simulink model "UNIFIER_3DOFsim"  (R2023b)
settings: Solver=VariableStepAuto  StartTime=0  StopTime=t_sim  RelTol=1e-3
InitFcn:
  | UNIFIER_3DOFsim_init
values from neighbouring files (symbols this model uses):
  b = 20.11467    [UNIFIER_LOAD.m]    (also in UNIFIER_LOAD.mat; UNIFIER_LOAD_ROM.m; UNIFIER_LOAD_ROM.mat)
  c = 1.43676    [UNIFIER_LOAD.m]    (also in UNIFIER_LOAD.mat; UNIFIER_LOAD_ROM.m; UNIFIER_LOAD_ROM.mat)
  DEP_inc = -0.0872664625997    [UNIFIER_LOAD.mat]    (also in UNIFIER_ROMdyn.m = deg2rad(-5); UNIFIER_ROMdyn_script.m = deg2rad(-5); UNIFIER_ROMdyn_v2.m = deg2rad(-5); UNIFIER_ROMgen.m = 0.1)
  dp_DEP =     [UNIFIER_LOAD.mat]    (also in UNIFIER_LOAD_ROM.mat)
  dp_FUSE_FIN =     [UNIFIER_LOAD.mat]
  dp_HTU =     [UNIFIER_LOAD.mat]    (also in UNIFIER_LOAD_ROM.mat)
  dp_VTAIL =     [UNIFIER_LOAD.mat]
  dp_VTAIL_INDUCED =     [UNIFIER_LOAD.mat]
  dp_WING_root =     [UNIFIER_LOAD.mat]
  dp_WING_tip =     [UNIFIER_LOAD.mat]
  dumax = [2.09439510239 2.09439510239 2.09439510239 1.0471975512 2 4 2]    [UNIFIER_LOAD.mat]    (also in UNIFIER_LOAD_ROM.mat = [1.0471975512 1.0471975512 1.0471975512 0.174532925199 2 2 2)
  gr = 9.80665    [UNIFIER_LOAD.mat]    (also in UNIFIER_LOAD_ROM.mat)
  m = 7057    [UNIFIER_LOAD.m]    (also in UNIFIER_LOAD.mat; UNIFIER_LOAD_ROM.m; UNIFIER_LOAD_ROM.mat)
  n_prop = 12    [UNIFIER_LOAD.mat]    (also in UNIFIER_ROMdyn.m; UNIFIER_ROMdyn_script.m; UNIFIER_ROMdyn_v2.m)
  prop_d = 1.6    [UNIFIER_LOAD.mat]    (also in UNIFIER_ROMdyn.m; UNIFIER_ROMdyn_script.m; UNIFIER_ROMdyn_v2.m)
  ROMv1 = ROM    [UNIFIER_3DOFsim_init.m]    (also in UNIFIER_ROMgen_subset.m; UNIFIER_ROMgen_v2_subset.m; UNIFIER_ROMgen_v3_subset.m; UNIFIER_ROMgen_v4_subset.m)
  ROMv2 = ROM    [UNIFIER_3DOFsim_init.m]
  ROMv3 = ROM    [UNIFIER_3DOFsim_init.m]
  S = 29.98388    [UNIFIER_LOAD.m]    (also in UNIFIER_LOAD.mat; UNIFIER_LOAD_ROM.m; UNIFIER_LOAD_ROM.mat)
  U_trim = [ustar(3) ... (first row only)    [UNIFIER_3DOFsim_init.m]
  umax = inf    [UNIFIERLanding.m]    (also in UNIFIER_LOAD.mat = [0.436332312999 0.523598775598 0.523598775598 0.436332312999; UNIFIER_LOAD_ROM.mat = [0.436332312999 0.523598775598 0.349065850399 0.436332312999)
  umin = 0    [UNIFIERLanding.m]    (also in UNIFIER_LOAD.mat = [-0.436332312999 -0.523598775598 -0.523598775598 0 0 -1 -0.5; UNIFIER_LOAD_ROM.mat = [-0.436332312999 -0.523598775598 -0.0872664625997 0 0 -1 0])
  Va = sqrt(u^2+w^2)    [ROMcomp.m]    (also in UNIFIERLanding.m = sqrt(x(:,3).^2+x(:,4).^2); UNIFIERLanding_Dynamics_Internal.m = sqrt(X(:,3).^2+X(:,4).^2); UNIFIERLanding_Main.m = sqrt(solution.X(:,3).^2+solution.X(:,4).^2); UNIFIERLanding_trajopt.m = sqrt(solution.X(:,3).^2+solution.X(:,4).^2))
  vtail_nodes = [dp_VTAIL.Xs_LE;     dp_VTAIL.Ys_LE;     dp_VTAIL.Zs_LE]    [UNIFIER_LOAD.m]    (also in UNIFIER_LOAD.mat = [-16.4894695282 -2.83441376686 -2.73765826225 -16.1370849609)
  wing_nodes = [fliplr(dp_WING_tip.LE_Xs),fliplr(dp_WING_root.LE_Xs),dp_WING_root.LE_Xs,dp_WING_tip.LE_Xs;     fliplr(-dp_WING_tip.LE_Ys),fliplr(-dp_WING_root.LE_Ys),dp_WING_root.LE_Ys,dp_WING_tip.LE_Ys;     fliplr(dp_WING_tip.LE_Zs),fliplr(dp_WING_root.LE_Zs),dp_WING_root.LE_Zs,dp_WING_tip.LE_Zs]    [UNIFIER_LOAD.m]    (also in UNIFIER_LOAD.mat = [-7.70795631409 -9.67500019073 -0.98178178072 -7.66801691055)
  x0 = xstar(1)    [UNIFIERLanding.m]    (also in UNIFIER_3DOFsim_init.m; UNIFIER_dynamics.m = x; UNIFIER_trim.m = [Va_target/100; UNIFIER_trim1.m = [Va_target)
  xstar = [0;        0;        -ze_target;        zstar(1)*100;        0;        zstar(2)*100;        0;        zstar(3);        0;        0;        0;        0]    [UNIFIER_trim.m]    (also in UNIFIER_trim0_res.mat = [0 0 -500 55.1327882403 0 -0.446351795968 0 1.36591182427e-0; UNIFIER_trim1.m = [0;        0;        -ze_target;        zstar(1);        0; ; UNIFIER_trim1_res.mat = [0 0 -1219 72.7310470326 0 1.14230710452 0 0.0157060522827 0; UNIFIER_trimHFM.m = [0;        0;        -runconfig.ze;        zstar(1)*100;    )
  xyz_cg = [-8.09,0,-0.2]    [UNIFIER_LOAD.m]    (also in UNIFIER_LOAD.mat = [-8.09 0 -0.2]; UNIFIER_LOAD_ROM.m; UNIFIER_LOAD_ROM.mat = [-8.09 0 -0.2])
  xyz_cg_12 = [-8.09 0 -0.2 -8.09 0 -0.2 -8.09 0 -0.2 -8.09 0 -0.2 ... (36 elements, 3x12)]    [UNIFIER_LOAD.mat]    (also in UNIFIER_LOAD_ROM.mat)
  xyz_DEP = [ -6.9629998	-6.9210000	-6.8660002	-6.8099999	-6.7540002	-6.6999998	-6.6999998	-6.7540002	-6.8099999	-6.8660002	-6.9210000	-6.9629998 ... (first row only)    [UNIFIER_LOAD.m]    (also in UNIFIER_LOAD.mat = [-6.9629998 -10.05 -0.90899998 -6.921 -8.4499998 -0.792 -6.8; UNIFIER_LOAD_ROM.m; UNIFIER_LOAD_ROM.mat = [-6.9629998 -10.05 -0.90899998 -6.921 -8.4499998 -0.792 -6.8)
  z0 = x(1,2)    [UNIFIERLanding.m]    (also in UNIFIER_3DOFsim_init.m = xstar(3); UNIFIER_trim.m = zstar; UNIFIER_trim1.m = zstar; UNIFIER_trimHFM.m = zstar)
undefined symbols (not defined in the file or in its folder): solution
libraries: simulink_extras x17, sharedutil x5, slpidlib x4, aerolibtransform2 x4, dspindex x2, matrix_library x1, shared6dof x1, aerolibatmos2 x1, simulink x1
(part 3 of 4)

== system UNIFIER_3DOFsim/UNIFIER/Aerodynamics/HFM/Aero/VtailForces/VtailForces ==
  rude_defl_nodes : Inport
  alpha_nodes : Inport  Port=2
  beta_nodes : Inport  Port=3
  Interpolation Using Prelookup1 : Interpolation_n-D  NumberOfTableDimensions=4  Table=dp_VTAIL.CFx  NumSelectionDims=1  InternalRulePriority=Speed  TableDataTypeStr=Inherit: Inherit from 'Table data'
      settings: InputPortMap=u0,u1,u2,u3,u4,u5,u6
  Interpolation Using Prelookup2 : Interpolation_n-D  NumberOfTableDimensions=4  Table=dp_VTAIL.CFy  NumSelectionDims=1  InternalRulePriority=Speed  TableDataTypeStr=Inherit: Inherit from 'Table data'
      settings: InputPortMap=u0,u1,u2,u3,u4,u5,u6
  Interpolation Using Prelookup3 : Interpolation_n-D  NumberOfTableDimensions=4  Table=dp_VTAIL.CFz  NumSelectionDims=1  InternalRulePriority=Speed  TableDataTypeStr=Inherit: Inherit from 'Table data'
      settings: InputPortMap=u0,u1,u2,u3,u4,u5,u6
  Interpolation Using Prelookup4 : Interpolation_n-D  NumberOfTableDimensions=4  Table=dp_VTAIL.CMx  NumSelectionDims=1  InternalRulePriority=Speed  TableDataTypeStr=Inherit: Inherit from 'Table data'
      settings: InputPortMap=u0,u1,u2,u3,u4,u5,u6
  Interpolation Using Prelookup5 : Interpolation_n-D  NumberOfTableDimensions=4  Table=dp_VTAIL.CMy  NumSelectionDims=1  InternalRulePriority=Speed  TableDataTypeStr=Inherit: Inherit from 'Table data'
      settings: InputPortMap=u0,u1,u2,u3,u4,u5,u6
  Interpolation Using Prelookup6 : Interpolation_n-D  NumberOfTableDimensions=4  Table=dp_VTAIL.CMz  NumSelectionDims=1  InternalRulePriority=Speed  TableDataTypeStr=Inherit: Inherit from 'Table data'
      settings: InputPortMap=u0,u1,u2,u3,u4,u5,u6
  WingRootPreLookup : Subsystem
  Cx : Outport
  Cy : Outport  Port=2
  Cz : Outport  Port=3
  CMx : Outport  Port=4
  CMy : Outport  Port=5
  CMz : Outport  Port=6
  wires:
  WingRootPreLookup/1(Out1) -> Interpolation Using Prelookup1/1, Interpolation Using Prelookup2/1, Interpolation Using Prelookup3/1, Interpolation Using Prelookup4/1, Interpolation Using Prelookup5/1, Interpolation Using Prelookup6/1
  Interpolation Using Prelookup6/1 -> CMz/1
  Interpolation Using Prelookup5/1 -> CMy/1
  Interpolation Using Prelookup4/1 -> CMx/1
  Interpolation Using Prelookup3/1 -> Cz/1
  Interpolation Using Prelookup2/1 -> Cy/1
  WingRootPreLookup/7(Out5) -> Interpolation Using Prelookup1/7, Interpolation Using Prelookup2/7, Interpolation Using Prelookup3/7, Interpolation Using Prelookup4/7, Interpolation Using Prelookup6/7, Interpolation Using Prelookup5/7
  alpha_nodes/1 -> WingRootPreLookup/2(alpha_nodes)
  beta_nodes/1 -> WingRootPreLookup/3(beta_nodes)
  WingRootPreLookup/2(Out2) -> Interpolation Using Prelookup1/2, Interpolation Using Prelookup2/2, Interpolation Using Prelookup3/2, Interpolation Using Prelookup6/2, Interpolation Using Prelookup5/2, Interpolation Using Prelookup4/2
  WingRootPreLookup/6(Out7) -> Interpolation Using Prelookup1/6, Interpolation Using Prelookup2/6, Interpolation Using Prelookup3/6, Interpolation Using Prelookup4/6, Interpolation Using Prelookup5/6, Interpolation Using Prelookup6/6
  Interpolation Using Prelookup1/1 -> Cx/1
  WingRootPreLookup/5(Out6) -> Interpolation Using Prelookup1/5, Interpolation Using Prelookup2/5, Interpolation Using Prelookup3/5, Interpolation Using Prelookup5/5, Interpolation Using Prelookup6/5, Interpolation Using Prelookup4/5
  WingRootPreLookup/4(Out4) -> Interpolation Using Prelookup1/4, Interpolation Using Prelookup2/4, Interpolation Using Prelookup3/4, Interpolation Using Prelookup4/4, Interpolation Using Prelookup5/4, Interpolation Using Prelookup6/4
  rude_defl_nodes/1 -> WingRootPreLookup/1(rude_defl_nodes)
  WingRootPreLookup/3(Out3) -> Interpolation Using Prelookup1/3, Interpolation Using Prelookup3/3, Interpolation Using Prelookup4/3, Interpolation Using Prelookup5/3, Interpolation Using Prelookup6/3, Interpolation Using Prelookup2/3

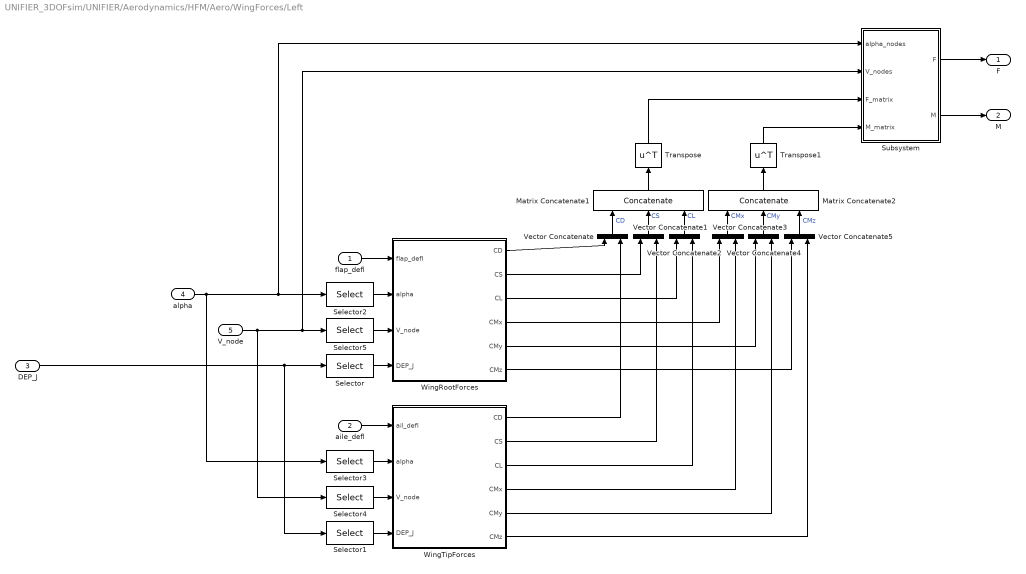
== system UNIFIER_3DOFsim/UNIFIER/Aerodynamics/HFM/Aero/WingForces/Left ==
  flap_defl : Inport
  aile_defl : Inport  Port=2
  DEP_J : Inport  Port=3  PortDimensions=6
  alpha : Inport  Port=4  PortDimensions=7
  V_node : Inport  Port=5  PortDimensions=7
  Matrix Concatenate1 : Concatenate  NumInputs=3  Mode=Multidimensional array  ConcatenateDimension=2
  Matrix Concatenate2 : Concatenate  NumInputs=3  Mode=Multidimensional array  ConcatenateDimension=2
  Selector : Selector  InputPortWidth=6  IndexOptions=Index vector (dialog)  Indices=[1,2,3,4,5]  OutputSizes=1
  Selector1 : Selector  InputPortWidth=6  IndexOptions=Index vector (dialog)  Indices=[5,6]  OutputSizes=1
  Selector2 : Selector  InputPortWidth=7  IndexOptions=Index vector (dialog)  Indices=[1,2,3,4,5]  OutputSizes=1
  Selector3 : Selector  InputPortWidth=7  IndexOptions=Index vector (dialog)  Indices=[6,7]  OutputSizes=1
  Selector4 : Selector  InputPortWidth=7  IndexOptions=Index vector (dialog)  Indices=[6,7]  OutputSizes=1
  Selector5 : Selector  InputPortWidth=7  IndexOptions=Index vector (dialog)  Indices=[1,2,3,4,5]  OutputSizes=1
  Subsystem : Subsystem
  Transpose : Math  Operator=transpose
  Transpose1 : Math  Operator=transpose
  Vector Concatenate{,1..5} (6 alike) : Concatenate
  WingRootForces : Subsystem
  WingTipForces : Subsystem
  F : Outport
  M : Outport  Port=2
  wires:
  Subsystem/2(M) -> M/1
  Subsystem/1(F) -> F/1
  Transpose1/1 -> Subsystem/4(M_matrix)
  Transpose/1 -> Subsystem/3(F_matrix)
  Matrix Concatenate2/1 -> Transpose1/1
  Vector Concatenate5/1 -> Matrix Concatenate2/3  "CMz"
  Vector Concatenate4/1 -> Matrix Concatenate2/2  "CMy"
  Vector Concatenate3/1 -> Matrix Concatenate2/1  "CMx"
  Vector Concatenate2/1 -> Matrix Concatenate1/3  "CL"
  Vector Concatenate/1 -> Matrix Concatenate1/1  "CD"
  Matrix Concatenate1/1 -> Transpose/1
  Vector Concatenate1/1 -> Matrix Concatenate1/2  "CS"
  WingRootForces/5(CMy) -> Vector Concatenate4/1
  WingRootForces/4(CMx) -> Vector Concatenate3/1
  WingRootForces/3(CL) -> Vector Concatenate2/1
  WingRootForces/2(CS) -> Vector Concatenate1/1
  Selector5/1 -> WingRootForces/3(V_node)
  Selector4/1 -> WingTipForces/3(V_node)
  Selector3/1 -> WingTipForces/2(alpha)
  Selector2/1 -> WingRootForces/2(alpha)
  aile_defl/1 -> WingTipForces/1(ail_defl)
  WingTipForces/4(CMx) -> Vector Concatenate3/2
  WingTipForces/5(CMy) -> Vector Concatenate4/2
  WingTipForces/3(CL) -> Vector Concatenate2/2
  WingTipForces/2(CS) -> Vector Concatenate1/2
  WingTipForces/6(CMz) -> Vector Concatenate5/2
  WingTipForces/1(CD) -> Vector Concatenate/2
  WingRootForces/6(CMz) -> Vector Concatenate5/1
  Selector1/1 -> WingTipForces/4(DEP_J)
  WingRootForces/1(CD) -> Vector Concatenate/1
  V_node/1 -> Selector5/1, Subsystem/2(V_nodes), Selector4/1
  Selector/1 -> WingRootForces/4(DEP_J)
  DEP_J/1 -> Selector/1, Selector1/1
  alpha/1 -> Selector3/1, Selector2/1, Subsystem/1(alpha_nodes)
  flap_defl/1 -> WingRootForces/1(flap_defl)

== system UNIFIER_3DOFsim/UNIFIER/Aerodynamics/HFM/Aero/WingForces/Right ==
  flap_defl : Inport
  aile_defl : Inport  Port=2
  DEP_J : Inport  Port=3  PortDimensions=6
  alpha : Inport  Port=4  PortDimensions=7
  V_node : Inport  Port=5  PortDimensions=7
  Matrix Concatenate1 : Concatenate  NumInputs=3  Mode=Multidimensional array  ConcatenateDimension=2
  Matrix Concatenate2 : Concatenate  NumInputs=3  Mode=Multidimensional array  ConcatenateDimension=2
  Selector : Selector  InputPortWidth=6  IndexOptions=Index vector (dialog)  Indices=[1,2,3,4,5]  OutputSizes=1
  Selector1 : Selector  InputPortWidth=6  IndexOptions=Index vector (dialog)  Indices=[5,6]  OutputSizes=1
  Selector2 : Selector  InputPortWidth=7  IndexOptions=Index vector (dialog)  Indices=[1,2,3,4,5]  OutputSizes=1
  Selector3 : Selector  InputPortWidth=7  IndexOptions=Index vector (dialog)  Indices=[6,7]  OutputSizes=1
  Selector4 : Selector  InputPortWidth=7  IndexOptions=Index vector (dialog)  Indices=[6,7]  OutputSizes=1
  Selector5 : Selector  InputPortWidth=7  IndexOptions=Index vector (dialog)  Indices=[1,2,3,4,5]  OutputSizes=1
  Subsystem : Subsystem
  Transpose : Math  Operator=transpose
  Transpose1 : Math  Operator=transpose
  Vector Concatenate{,1..5} (6 alike) : Concatenate
  WingRootForces : Subsystem
  WingTipForces : Subsystem
  F : Outport
  M : Outport  Port=2
  wires:
  Subsystem/2(M) -> M/1
  Subsystem/1(F) -> F/1
  Transpose1/1 -> Subsystem/4(M_matrix)
  Transpose/1 -> Subsystem/3(F_matrix)
  Matrix Concatenate2/1 -> Transpose1/1
  Vector Concatenate5/1 -> Matrix Concatenate2/3  "CMz"
  Vector Concatenate4/1 -> Matrix Concatenate2/2  "CMy"
  Vector Concatenate3/1 -> Matrix Concatenate2/1  "CMx"
  Vector Concatenate2/1 -> Matrix Concatenate1/3  "CL"
  Vector Concatenate/1 -> Matrix Concatenate1/1  "CD"
  Matrix Concatenate1/1 -> Transpose/1
  Vector Concatenate1/1 -> Matrix Concatenate1/2  "CS"
  WingRootForces/5(CMy) -> Vector Concatenate4/1
  WingRootForces/4(CMx) -> Vector Concatenate3/1
  WingRootForces/3(CL) -> Vector Concatenate2/1
  WingRootForces/2(CS) -> Vector Concatenate1/1
  Selector5/1 -> WingRootForces/3(V_node)
  Selector4/1 -> WingTipForces/3(V_node)
  Selector3/1 -> WingTipForces/2(alpha)
  Selector2/1 -> WingRootForces/2(alpha)
  aile_defl/1 -> WingTipForces/1(ail_defl)
  WingTipForces/4(CMx) -> Vector Concatenate3/2
  WingTipForces/5(CMy) -> Vector Concatenate4/2
  WingTipForces/3(CL) -> Vector Concatenate2/2
  WingTipForces/2(CS) -> Vector Concatenate1/2
  WingTipForces/6(CMz) -> Vector Concatenate5/2
  WingTipForces/1(CD) -> Vector Concatenate/2
  WingRootForces/6(CMz) -> Vector Concatenate5/1
  Selector1/1 -> WingTipForces/4(DEP_J)
  WingRootForces/1(CD) -> Vector Concatenate/1
  V_node/1 -> Selector5/1, Subsystem/2(V_nodes), Selector4/1
  Selector/1 -> WingRootForces/4(DEP_J)
  DEP_J/1 -> Selector/1, Selector1/1
  alpha/1 -> Selector3/1, Selector2/1, Subsystem/1(alpha_nodes)
  flap_defl/1 -> WingRootForces/1(flap_defl)

== system UNIFIER_3DOFsim/UNIFIER/Aerodynamics/HFM/Aero/WingForces/Subsystem ==
  DEP_J : Inport
  alpha_nodes : Inport  Port=2
  V_nodes : Inport  Port=3
  Demux1 : Demux  Outputs=2
  Demux2 : Demux  Outputs=2
  Demux3 : Demux  Outputs=2
  Selector : Selector  InputPortWidth=6  IndexOptions=Index vector (dialog)  Indices=[6,5,4,3,2,1]  OutputSizes=1
  Selector1 : Selector  InputPortWidth=7  IndexOptions=Index vector (dialog)  Indices=[7,6,5,4,3,2,1]  OutputSizes=1
  Selector2 : Selector  InputPortWidth=7  IndexOptions=Index vector (dialog)  Indices=[7,6,5,4,3,2,1]  OutputSizes=1
  DEP_J_Left : Outport  PortDimensions=6
  alpha_nodes_Left : Outport  Port=2  PortDimensions=7
  V_nodes_Left : Outport  Port=3  PortDimensions=7
  DEP_J_Right : Outport  Port=4  PortDimensions=6
  alpha_nodes_Right : Outport  Port=5  PortDimensions=7
  V_nodes_Right : Outport  Port=6  PortDimensions=7
  wires:
  Demux3/2 -> V_nodes_Right/1
  V_nodes/1 -> Demux3/1
  Selector2/1 -> V_nodes_Left/1
  Demux3/1 -> Selector2/1
  Demux1/1 -> Selector1/1
  Demux1/2 -> alpha_nodes_Right/1
  alpha_nodes/1 -> Demux1/1
  Selector1/1 -> alpha_nodes_Left/1
  Selector/1 -> DEP_J_Left/1
  DEP_J/1 -> Demux2/1
  Demux2/1 -> Selector/1
  Demux2/2 -> DEP_J_Right/1

== system UNIFIER_3DOFsim/UNIFIER/Aerodynamics/HFM/Aero/FinFuselageForces/Subsystem1/Subsystem ==
  beta : Inport
  alpha : Inport  Port=2
  Prelookup : PreLookup  BreakpointsData=dp_FUSE_FIN.beta  IndexSearchMethod=Linear search  BeginIndexSearchUsingPreviousIndexResult=on  ExtrapMethod=Linear
  Prelookup1 : PreLookup  BreakpointsData=dp_FUSE_FIN.aoa  IndexSearchMethod=Linear search  BeginIndexSearchUsingPreviousIndexResult=on  ExtrapMethod=Linear
  Out1 : Outport
  Out2 : Outport  Port=2
  Out3 : Outport  Port=3
  Out4 : Outport  Port=4
  wires:
  Prelookup/2 -> Out2/1
  Prelookup1/2 -> Out4/1
  Prelookup1/1 -> Out3/1
  beta/1 -> Prelookup/1
  alpha/1 -> Prelookup1/1
  Prelookup/1 -> Out1/1

== system UNIFIER_3DOFsim/UNIFIER/Aerodynamics/HFM/Aero/VtailForces/Subsystem/CrossProduct1 ==
  r : Inport  Partition=on  PartitionDimension=2  PartitionWidth=1  PartitionOffset=0
  F : Inport  Port=2  Partition=on  PartitionDimension=2  PartitionWidth=1  PartitionOffset=0
  3x3 Cross Product : sharedutil/3x3 Cross Product  aMode=aMode
  CG : Constant  Value=xyz_cg
  Cast : DataTypeConversion  OutDataTypeStr=single  SaturateOnIntegerOverflow=off  RndMeth=Floor
  For Each : ForEach  DisableCoverage=on  SpecifiedNumIters=16
  Minus : Sum  Inputs=+-
  M : Outport  ConcatenationDimension=2
  wires:
  Cast/1 -> Minus/2
  Minus/1 -> 3x3 Cross Product/1
  CG/1 -> Cast/1
  3x3 Cross Product/1 -> M/1
  r/1 -> Minus/1
  F/1 -> 3x3 Cross Product/2

== system UNIFIER_3DOFsim/UNIFIER/Aerodynamics/HFM/Aero/VtailForces/VtailForces/WingRootPreLookup ==
  rude_defl_nodes : Inport
  alpha_nodes : Inport  Port=2
  beta_nodes : Inport  Port=3
  Constant8 : Constant  Value=0:15
  Prelookup : PreLookup  BreakpointsData=dp_VTAIL.rude_defl  IndexSearchMethod=Linear search  BeginIndexSearchUsingPreviousIndexResult=on  ExtrapMethod=Linear
  Prelookup1 : PreLookup  BreakpointsData=dp_VTAIL.alphas  IndexSearchMethod=Linear search  BeginIndexSearchUsingPreviousIndexResult=on  ExtrapMethod=Linear
  Prelookup2 : PreLookup  BreakpointsData=dp_VTAIL.betas  IndexSearchMethod=Linear search  BeginIndexSearchUsingPreviousIndexResult=on  ExtrapMethod=Linear
  Out1 : Outport
  Out2 : Outport  Port=2
  Out3 : Outport  Port=3
  Out4 : Outport  Port=4
  Out6 : Outport  Port=5
  Out7 : Outport  Port=6
  Out5 : Outport  Port=7
  wires:
  Prelookup2/2 -> Out7/1
  Prelookup2/1 -> Out6/1
  beta_nodes/1 -> Prelookup2/1
  rude_defl_nodes/1 -> Prelookup/1
  Prelookup1/1 -> Out3/1
  alpha_nodes/1 -> Prelookup1/1
  Prelookup/2 -> Out2/1
  Prelookup1/2 -> Out4/1
  Constant8/1 -> Out5/1
  Prelookup/1 -> Out1/1

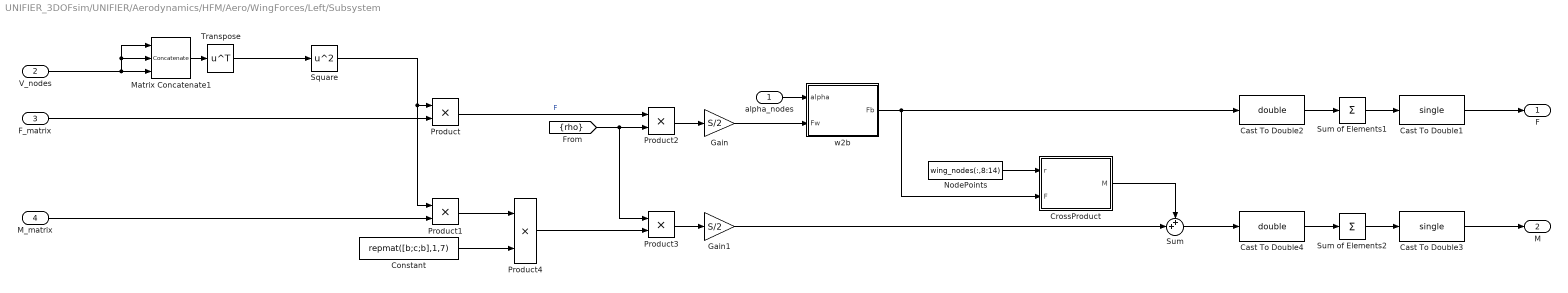
== system UNIFIER_3DOFsim/UNIFIER/Aerodynamics/HFM/Aero/WingForces/Left/Subsystem ==
  alpha_nodes : Inport
  V_nodes : Inport  Port=2
  F_matrix : Inport  Port=3
  M_matrix : Inport  Port=4
  Cast To Double1 : DataTypeConversion  OutDataTypeStr=single  SaturateOnIntegerOverflow=off  RndMeth=Floor
  Cast To Double2 : DataTypeConversion  OutDataTypeStr=double  SaturateOnIntegerOverflow=off  RndMeth=Floor
  Cast To Double3 : DataTypeConversion  OutDataTypeStr=single  SaturateOnIntegerOverflow=off  RndMeth=Floor
  Cast To Double4 : DataTypeConversion  OutDataTypeStr=double  SaturateOnIntegerOverflow=off  RndMeth=Floor
  Constant : Constant  Value=repmat([b;c;b],1,7)
  CrossProduct : Subsystem  TreatAsAtomicUnit=on
  Gain : Gain  Gain=S/2
  Gain1 : Gain  Gain=S/2
  Matrix Concatenate1 : Concatenate  NumInputs=3  Mode=Multidimensional array  ConcatenateDimension=2
  NodePoints : Constant  Value=wing_nodes(:,8:14)
  Product{,1..4} (5 alike) : Product
  Square : Math  Operator=square
  Sum : Sum  Inputs=++|
  Sum of Elements1 : Sum  Inputs=+  CollapseMode=Specified dimension  CollapseDim=2
  Sum of Elements2 : Sum  Inputs=+  CollapseMode=Specified dimension  CollapseDim=2
  Transpose : Math  Operator=transpose
  w2b : Subsystem  TreatAsAtomicUnit=on
  F : Outport
  M : Outport  Port=2
  wires:
  Cast To Double3/1 -> M/1
  Sum/1 -> Cast To Double4/1
  Cast To Double4/1 -> Sum of Elements2/1
  Sum of Elements2/1 -> Cast To Double3/1
  Sum of Elements1/1 -> Cast To Double1/1
  Cast To Double2/1 -> Sum of Elements1/1
  alpha_nodes/1 -> w2b/1(alpha)
  Gain/1 -> w2b/2(Fw)
  Cast To Double1/1 -> F/1
  CrossProduct/1(M) -> Sum/1
  NodePoints/1 -> CrossProduct/1(r)
  w2b/1(Fb) -> CrossProduct/2(F), Cast To Double2/1
  Square/1 -> Product/1, Product1/1
  Matrix Concatenate1/1 -> Transpose/1
  Transpose/1 -> Square/1
  V_nodes/1 -> Matrix Concatenate1/3, Matrix Concatenate1/2, Matrix Concatenate1/1
  Product/1 -> Product2/1  "F"
  Gain1/1 -> Sum/2
  Product1/1 -> Product4/1
  M_matrix/1 -> Product1/2
  Product4/1 -> Product3/2
  Constant/1 -> Product4/2
  Product3/1 -> Gain1/1
  [rho] -> Product2/2, Product3/1
  F_matrix/1 -> Product/2
  Product2/1 -> Gain/1

== system UNIFIER_3DOFsim/UNIFIER/Aerodynamics/HFM/Aero/WingForces/Left/WingRootForces ==
  flap_defl : Inport
  alpha : Inport  Port=2
  V_node : Inport  Port=3
  DEP_J : Inport  Port=4
  Interpolation Using Prelookup1 : Interpolation_n-D  NumberOfTableDimensions=5  Table=dp_WING_root.CD  ExtrapMethod=Clip  ValidIndexMayReachLast=on  NumSelectionDims=1  InternalRulePriority=Speed  TableDataTypeStr=Inherit: Inherit from 'Table data'
      settings: InputPortMap=u0,u1,u2,u3,u4,u5,u6,u7,u8
  Interpolation Using Prelookup2 : Interpolation_n-D  NumberOfTableDimensions=5  Table=dp_WING_root.CS  ExtrapMethod=Clip  ValidIndexMayReachLast=on  NumSelectionDims=1  InternalRulePriority=Speed  TableDataTypeStr=Inherit: Inherit from 'Table data'
      settings: InputPortMap=u0,u1,u2,u3,u4,u5,u6,u7,u8
  Interpolation Using Prelookup3 : Interpolation_n-D  NumberOfTableDimensions=5  Table=dp_WING_root.CL  ExtrapMethod=Clip  ValidIndexMayReachLast=on  NumSelectionDims=1  InternalRulePriority=Speed  TableDataTypeStr=Inherit: Inherit from 'Table data'
      settings: InputPortMap=u0,u1,u2,u3,u4,u5,u6,u7,u8
  Interpolation Using Prelookup4 : Interpolation_n-D  NumberOfTableDimensions=5  Table=dp_WING_root.CMx  ExtrapMethod=Clip  ValidIndexMayReachLast=on  NumSelectionDims=1  InternalRulePriority=Speed  TableDataTypeStr=Inherit: Inherit from 'Table data'
      settings: InputPortMap=u0,u1,u2,u3,u4,u5,u6,u7,u8
  Interpolation Using Prelookup5 : Interpolation_n-D  NumberOfTableDimensions=5  Table=dp_WING_root.CMy  ExtrapMethod=Clip  ValidIndexMayReachLast=on  NumSelectionDims=1  InternalRulePriority=Speed  TableDataTypeStr=Inherit: Inherit from 'Table data'
      settings: InputPortMap=u0,u1,u2,u3,u4,u5,u6,u7,u8
  Interpolation Using Prelookup6 : Interpolation_n-D  NumberOfTableDimensions=5  Table=dp_WING_root.CMz  ExtrapMethod=Clip  ValidIndexMayReachLast=on  NumSelectionDims=1  InternalRulePriority=Speed  TableDataTypeStr=Inherit: Inherit from 'Table data'
      settings: InputPortMap=u0,u1,u2,u3,u4,u5,u6,u7,u8
  WingRootPreLookup : Subsystem
  CD : Outport
  CS : Outport  Port=2
  CL : Outport  Port=3
  CMx : Outport  Port=4
  CMy : Outport  Port=5
  CMz : Outport  Port=6
  wires:
  Interpolation Using Prelookup6/1 -> CMz/1
  Interpolation Using Prelookup5/1 -> CMy/1
  Interpolation Using Prelookup4/1 -> CMx/1
  Interpolation Using Prelookup3/1 -> CL/1
  Interpolation Using Prelookup2/1 -> CS/1
  alpha/1 -> WingRootPreLookup/2(alpha)
  V_node/1 -> WingRootPreLookup/3(V_node)
  DEP_J/1 -> WingRootPreLookup/4(DEP_J)
  WingRootPreLookup/2(Out2) -> Interpolation Using Prelookup1/2, Interpolation Using Prelookup2/2, Interpolation Using Prelookup3/2, Interpolation Using Prelookup4/2, Interpolation Using Prelookup5/2, Interpolation Using Prelookup6/2
  WingRootPreLookup/6(Out7) -> Interpolation Using Prelookup1/6, Interpolation Using Prelookup2/6, Interpolation Using Prelookup3/6, Interpolation Using Prelookup4/6, Interpolation Using Prelookup5/6, Interpolation Using Prelookup6/6
  Interpolation Using Prelookup1/1 -> CD/1
  WingRootPreLookup/5(Out6) -> Interpolation Using Prelookup2/5, Interpolation Using Prelookup3/5, Interpolation Using Prelookup4/5, Interpolation Using Prelookup5/5, Interpolation Using Prelookup6/5, Interpolation Using Prelookup1/5
  WingRootPreLookup/4(Out4) -> Interpolation Using Prelookup1/4, Interpolation Using Prelookup2/4, Interpolation Using Prelookup3/4, Interpolation Using Prelookup4/4, Interpolation Using Prelookup5/4, Interpolation Using Prelookup6/4
  flap_defl/1 -> WingRootPreLookup/1(flap_defl)
  WingRootPreLookup/7(Out8) -> Interpolation Using Prelookup2/7, Interpolation Using Prelookup3/7, Interpolation Using Prelookup4/7, Interpolation Using Prelookup6/7, Interpolation Using Prelookup5/7, Interpolation Using Prelookup1/7
  WingRootPreLookup/1(Out1) -> Interpolation Using Prelookup1/1, Interpolation Using Prelookup2/1, Interpolation Using Prelookup3/1, Interpolation Using Prelookup4/1, Interpolation Using Prelookup5/1, Interpolation Using Prelookup6/1
  WingRootPreLookup/8(Out9) -> Interpolation Using Prelookup1/8, Interpolation Using Prelookup2/8, Interpolation Using Prelookup3/8, Interpolation Using Prelookup4/8, Interpolation Using Prelookup5/8, Interpolation Using Prelookup6/8
  WingRootPreLookup/3(Out3) -> Interpolation Using Prelookup1/3, Interpolation Using Prelookup2/3, Interpolation Using Prelookup3/3, Interpolation Using Prelookup4/3, Interpolation Using Prelookup5/3, Interpolation Using Prelookup6/3
  WingRootPreLookup/9(Out5) -> Interpolation Using Prelookup1/9, Interpolation Using Prelookup2/9, Interpolation Using Prelookup3/9, Interpolation Using Prelookup4/9, Interpolation Using Prelookup5/9, Interpolation Using Prelookup6/9

== system UNIFIER_3DOFsim/UNIFIER/Aerodynamics/HFM/Aero/WingForces/Left/WingTipForces ==
  ail_defl : Inport
  alpha : Inport  Port=2
  V_node : Inport  Port=3
  DEP_J : Inport  Port=4
  Interpolation Using Prelookup1 : Interpolation_n-D  NumberOfTableDimensions=5  Table=dp_WING_tip.CD  ExtrapMethod=Clip  ValidIndexMayReachLast=on  NumSelectionDims=1  InternalRulePriority=Speed  TableDataTypeStr=Inherit: Inherit from 'Table data'
      settings: InputPortMap=u0,u1,u2,u3,u4,u5,u6,u7,u8
  Interpolation Using Prelookup2 : Interpolation_n-D  NumberOfTableDimensions=5  Table=dp_WING_tip.CS  ExtrapMethod=Clip  ValidIndexMayReachLast=on  NumSelectionDims=1  InternalRulePriority=Speed  TableDataTypeStr=Inherit: Inherit from 'Table data'
      settings: InputPortMap=u0,u1,u2,u3,u4,u5,u6,u7,u8
  Interpolation Using Prelookup3 : Interpolation_n-D  NumberOfTableDimensions=5  Table=dp_WING_tip.CL  ExtrapMethod=Clip  ValidIndexMayReachLast=on  NumSelectionDims=1  InternalRulePriority=Speed  TableDataTypeStr=Inherit: Inherit from 'Table data'
      settings: InputPortMap=u0,u1,u2,u3,u4,u5,u6,u7,u8
  Interpolation Using Prelookup4 : Interpolation_n-D  NumberOfTableDimensions=5  Table=dp_WING_tip.CMx  ExtrapMethod=Clip  ValidIndexMayReachLast=on  NumSelectionDims=1  InternalRulePriority=Speed  TableDataTypeStr=Inherit: Inherit from 'Table data'
      settings: InputPortMap=u0,u1,u2,u3,u4,u5,u6,u7,u8
  Interpolation Using Prelookup5 : Interpolation_n-D  NumberOfTableDimensions=5  Table=dp_WING_tip.CMy  ExtrapMethod=Clip  ValidIndexMayReachLast=on  NumSelectionDims=1  InternalRulePriority=Speed  TableDataTypeStr=Inherit: Inherit from 'Table data'
      settings: InputPortMap=u0,u1,u2,u3,u4,u5,u6,u7,u8
  Interpolation Using Prelookup6 : Interpolation_n-D  NumberOfTableDimensions=5  Table=dp_WING_tip.CMz  ExtrapMethod=Clip  ValidIndexMayReachLast=on  NumSelectionDims=1  InternalRulePriority=Speed  TableDataTypeStr=Inherit: Inherit from 'Table data'
      settings: InputPortMap=u0,u1,u2,u3,u4,u5,u6,u7,u8
  WingRootPreLookup : Subsystem
  CD : Outport
  CS : Outport  Port=2
  CL : Outport  Port=3
  CMx : Outport  Port=4
  CMy : Outport  Port=5
  CMz : Outport  Port=6
  wires:
  Interpolation Using Prelookup6/1 -> CMz/1
  Interpolation Using Prelookup5/1 -> CMy/1
  Interpolation Using Prelookup4/1 -> CMx/1
  Interpolation Using Prelookup3/1 -> CL/1
  Interpolation Using Prelookup2/1 -> CS/1
  alpha/1 -> WingRootPreLookup/2(alpha)
  V_node/1 -> WingRootPreLookup/3(V_node)
  DEP_J/1 -> WingRootPreLookup/4(DEP_J)
  WingRootPreLookup/2(Out2) -> Interpolation Using Prelookup1/2, Interpolation Using Prelookup2/2, Interpolation Using Prelookup3/2, Interpolation Using Prelookup4/2, Interpolation Using Prelookup5/2, Interpolation Using Prelookup6/2
  WingRootPreLookup/6(Out7) -> Interpolation Using Prelookup1/6, Interpolation Using Prelookup2/6, Interpolation Using Prelookup3/6, Interpolation Using Prelookup4/6, Interpolation Using Prelookup5/6, Interpolation Using Prelookup6/6
  Interpolation Using Prelookup1/1 -> CD/1
  WingRootPreLookup/5(Out6) -> Interpolation Using Prelookup2/5, Interpolation Using Prelookup3/5, Interpolation Using Prelookup4/5, Interpolation Using Prelookup5/5, Interpolation Using Prelookup6/5, Interpolation Using Prelookup1/5
  WingRootPreLookup/4(Out4) -> Interpolation Using Prelookup1/4, Interpolation Using Prelookup2/4, Interpolation Using Prelookup3/4, Interpolation Using Prelookup4/4, Interpolation Using Prelookup5/4, Interpolation Using Prelookup6/4
  ail_defl/1 -> WingRootPreLookup/1(ail_defl)
  WingRootPreLookup/7(Out8) -> Interpolation Using Prelookup1/7, Interpolation Using Prelookup2/7, Interpolation Using Prelookup3/7, Interpolation Using Prelookup4/7, Interpolation Using Prelookup6/7, Interpolation Using Prelookup5/7
  WingRootPreLookup/1(Out1) -> Interpolation Using Prelookup1/1, Interpolation Using Prelookup2/1, Interpolation Using Prelookup3/1, Interpolation Using Prelookup4/1, Interpolation Using Prelookup5/1, Interpolation Using Prelookup6/1
  WingRootPreLookup/8(Out9) -> Interpolation Using Prelookup1/8, Interpolation Using Prelookup2/8, Interpolation Using Prelookup3/8, Interpolation Using Prelookup4/8, Interpolation Using Prelookup5/8, Interpolation Using Prelookup6/8
  WingRootPreLookup/3(Out3) -> Interpolation Using Prelookup1/3, Interpolation Using Prelookup2/3, Interpolation Using Prelookup3/3, Interpolation Using Prelookup4/3, Interpolation Using Prelookup5/3, Interpolation Using Prelookup6/3
  WingRootPreLookup/9(Out5) -> Interpolation Using Prelookup1/9, Interpolation Using Prelookup2/9, Interpolation Using Prelookup3/9, Interpolation Using Prelookup4/9, Interpolation Using Prelookup5/9, Interpolation Using Prelookup6/9

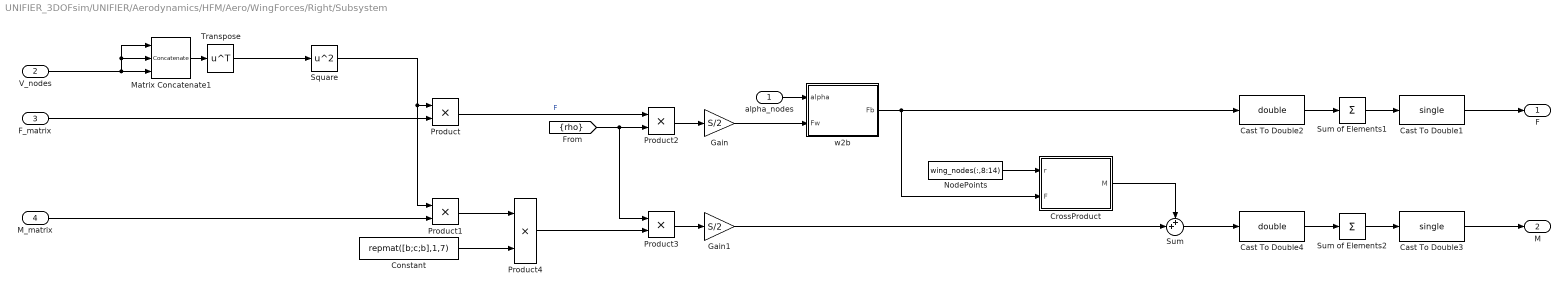
== system UNIFIER_3DOFsim/UNIFIER/Aerodynamics/HFM/Aero/WingForces/Right/Subsystem ==
  alpha_nodes : Inport
  V_nodes : Inport  Port=2
  F_matrix : Inport  Port=3
  M_matrix : Inport  Port=4
  Cast To Double1 : DataTypeConversion  OutDataTypeStr=single  SaturateOnIntegerOverflow=off  RndMeth=Floor
  Cast To Double2 : DataTypeConversion  OutDataTypeStr=double  SaturateOnIntegerOverflow=off  RndMeth=Floor
  Cast To Double3 : DataTypeConversion  OutDataTypeStr=single  SaturateOnIntegerOverflow=off  RndMeth=Floor
  Cast To Double4 : DataTypeConversion  OutDataTypeStr=double  SaturateOnIntegerOverflow=off  RndMeth=Floor
  Constant : Constant  Value=repmat([b;c;b],1,7)
  CrossProduct : Subsystem  TreatAsAtomicUnit=on
  Gain : Gain  Gain=S/2
  Gain1 : Gain  Gain=S/2
  Matrix Concatenate1 : Concatenate  NumInputs=3  Mode=Multidimensional array  ConcatenateDimension=2
  NodePoints : Constant  Value=wing_nodes(:,8:14)
  Product{,1..4} (5 alike) : Product
  Square : Math  Operator=square
  Sum : Sum  Inputs=++|
  Sum of Elements1 : Sum  Inputs=+  CollapseMode=Specified dimension  CollapseDim=2
  Sum of Elements2 : Sum  Inputs=+  CollapseMode=Specified dimension  CollapseDim=2
  Transpose : Math  Operator=transpose
  w2b : Subsystem  TreatAsAtomicUnit=on
  F : Outport
  M : Outport  Port=2
  wires:
  Cast To Double3/1 -> M/1
  Sum/1 -> Cast To Double4/1
  Cast To Double4/1 -> Sum of Elements2/1
  Sum of Elements2/1 -> Cast To Double3/1
  Sum of Elements1/1 -> Cast To Double1/1
  Cast To Double2/1 -> Sum of Elements1/1
  alpha_nodes/1 -> w2b/1(alpha)
  Gain/1 -> w2b/2(Fw)
  Cast To Double1/1 -> F/1
  CrossProduct/1(M) -> Sum/1
  NodePoints/1 -> CrossProduct/1(r)
  w2b/1(Fb) -> CrossProduct/2(F), Cast To Double2/1
  Square/1 -> Product/1, Product1/1
  Matrix Concatenate1/1 -> Transpose/1
  Transpose/1 -> Square/1
  V_nodes/1 -> Matrix Concatenate1/3, Matrix Concatenate1/2, Matrix Concatenate1/1
  Product/1 -> Product2/1  "F"
  Gain1/1 -> Sum/2
  Product1/1 -> Product4/1
  M_matrix/1 -> Product1/2
  Product4/1 -> Product3/2
  Constant/1 -> Product4/2
  Product3/1 -> Gain1/1
  [rho] -> Product2/2, Product3/1
  F_matrix/1 -> Product/2
  Product2/1 -> Gain/1

== system UNIFIER_3DOFsim/UNIFIER/Aerodynamics/HFM/Aero/WingForces/Right/WingRootForces ==
  flap_defl : Inport
  alpha : Inport  Port=2
  V_node : Inport  Port=3
  DEP_J : Inport  Port=4
  Interpolation Using Prelookup1 : Interpolation_n-D  NumberOfTableDimensions=5  Table=dp_WING_root.CD  ExtrapMethod=Clip  ValidIndexMayReachLast=on  NumSelectionDims=1  InternalRulePriority=Speed  TableDataTypeStr=Inherit: Inherit from 'Table data'
      settings: InputPortMap=u0,u1,u2,u3,u4,u5,u6,u7,u8
  Interpolation Using Prelookup2 : Interpolation_n-D  NumberOfTableDimensions=5  Table=dp_WING_root.CS  ExtrapMethod=Clip  ValidIndexMayReachLast=on  NumSelectionDims=1  InternalRulePriority=Speed  TableDataTypeStr=Inherit: Inherit from 'Table data'
      settings: InputPortMap=u0,u1,u2,u3,u4,u5,u6,u7,u8
  Interpolation Using Prelookup3 : Interpolation_n-D  NumberOfTableDimensions=5  Table=dp_WING_root.CL  ExtrapMethod=Clip  ValidIndexMayReachLast=on  NumSelectionDims=1  InternalRulePriority=Speed  TableDataTypeStr=Inherit: Inherit from 'Table data'
      settings: InputPortMap=u0,u1,u2,u3,u4,u5,u6,u7,u8
  Interpolation Using Prelookup4 : Interpolation_n-D  NumberOfTableDimensions=5  Table=dp_WING_root.CMx  ExtrapMethod=Clip  ValidIndexMayReachLast=on  NumSelectionDims=1  InternalRulePriority=Speed  TableDataTypeStr=Inherit: Inherit from 'Table data'
      settings: InputPortMap=u0,u1,u2,u3,u4,u5,u6,u7,u8
  Interpolation Using Prelookup5 : Interpolation_n-D  NumberOfTableDimensions=5  Table=dp_WING_root.CMy  ExtrapMethod=Clip  ValidIndexMayReachLast=on  NumSelectionDims=1  InternalRulePriority=Speed  TableDataTypeStr=Inherit: Inherit from 'Table data'
      settings: InputPortMap=u0,u1,u2,u3,u4,u5,u6,u7,u8
  Interpolation Using Prelookup6 : Interpolation_n-D  NumberOfTableDimensions=5  Table=dp_WING_root.CMz  ExtrapMethod=Clip  ValidIndexMayReachLast=on  NumSelectionDims=1  InternalRulePriority=Speed  TableDataTypeStr=Inherit: Inherit from 'Table data'
      settings: InputPortMap=u0,u1,u2,u3,u4,u5,u6,u7,u8
  WingRootPreLookup : Subsystem
  CD : Outport
  CS : Outport  Port=2
  CL : Outport  Port=3
  CMx : Outport  Port=4
  CMy : Outport  Port=5
  CMz : Outport  Port=6
  wires:
  Interpolation Using Prelookup6/1 -> CMz/1
  Interpolation Using Prelookup5/1 -> CMy/1
  Interpolation Using Prelookup4/1 -> CMx/1
  Interpolation Using Prelookup3/1 -> CL/1
  Interpolation Using Prelookup2/1 -> CS/1
  alpha/1 -> WingRootPreLookup/2(alpha)
  V_node/1 -> WingRootPreLookup/3(V_node)
  DEP_J/1 -> WingRootPreLookup/4(DEP_J)
  WingRootPreLookup/2(Out2) -> Interpolation Using Prelookup1/2, Interpolation Using Prelookup2/2, Interpolation Using Prelookup3/2, Interpolation Using Prelookup4/2, Interpolation Using Prelookup5/2, Interpolation Using Prelookup6/2
  WingRootPreLookup/6(Out7) -> Interpolation Using Prelookup1/6, Interpolation Using Prelookup2/6, Interpolation Using Prelookup3/6, Interpolation Using Prelookup4/6, Interpolation Using Prelookup5/6, Interpolation Using Prelookup6/6
  Interpolation Using Prelookup1/1 -> CD/1
  WingRootPreLookup/5(Out6) -> Interpolation Using Prelookup2/5, Interpolation Using Prelookup3/5, Interpolation Using Prelookup4/5, Interpolation Using Prelookup5/5, Interpolation Using Prelookup6/5, Interpolation Using Prelookup1/5
  WingRootPreLookup/4(Out4) -> Interpolation Using Prelookup1/4, Interpolation Using Prelookup2/4, Interpolation Using Prelookup3/4, Interpolation Using Prelookup4/4, Interpolation Using Prelookup5/4, Interpolation Using Prelookup6/4
  flap_defl/1 -> WingRootPreLookup/1(flap_defl)
  WingRootPreLookup/7(Out8) -> Interpolation Using Prelookup2/7, Interpolation Using Prelookup3/7, Interpolation Using Prelookup4/7, Interpolation Using Prelookup6/7, Interpolation Using Prelookup5/7, Interpolation Using Prelookup1/7
  WingRootPreLookup/1(Out1) -> Interpolation Using Prelookup1/1, Interpolation Using Prelookup2/1, Interpolation Using Prelookup3/1, Interpolation Using Prelookup4/1, Interpolation Using Prelookup5/1, Interpolation Using Prelookup6/1
  WingRootPreLookup/8(Out9) -> Interpolation Using Prelookup1/8, Interpolation Using Prelookup2/8, Interpolation Using Prelookup3/8, Interpolation Using Prelookup4/8, Interpolation Using Prelookup5/8, Interpolation Using Prelookup6/8
  WingRootPreLookup/3(Out3) -> Interpolation Using Prelookup1/3, Interpolation Using Prelookup2/3, Interpolation Using Prelookup3/3, Interpolation Using Prelookup4/3, Interpolation Using Prelookup5/3, Interpolation Using Prelookup6/3
  WingRootPreLookup/9(Out5) -> Interpolation Using Prelookup1/9, Interpolation Using Prelookup2/9, Interpolation Using Prelookup3/9, Interpolation Using Prelookup4/9, Interpolation Using Prelookup5/9, Interpolation Using Prelookup6/9

== system UNIFIER_3DOFsim/UNIFIER/Aerodynamics/HFM/Aero/WingForces/Right/WingTipForces ==
  ail_defl : Inport
  alpha : Inport  Port=2
  V_node : Inport  Port=3
  DEP_J : Inport  Port=4
  Interpolation Using Prelookup1 : Interpolation_n-D  NumberOfTableDimensions=5  Table=dp_WING_tip.CD  ExtrapMethod=Clip  ValidIndexMayReachLast=on  NumSelectionDims=1  InternalRulePriority=Speed  TableDataTypeStr=Inherit: Inherit from 'Table data'
      settings: InputPortMap=u0,u1,u2,u3,u4,u5,u6,u7,u8
  Interpolation Using Prelookup2 : Interpolation_n-D  NumberOfTableDimensions=5  Table=dp_WING_tip.CS  ExtrapMethod=Clip  ValidIndexMayReachLast=on  NumSelectionDims=1  InternalRulePriority=Speed  TableDataTypeStr=Inherit: Inherit from 'Table data'
      settings: InputPortMap=u0,u1,u2,u3,u4,u5,u6,u7,u8
  Interpolation Using Prelookup3 : Interpolation_n-D  NumberOfTableDimensions=5  Table=dp_WING_tip.CL  ExtrapMethod=Clip  ValidIndexMayReachLast=on  NumSelectionDims=1  InternalRulePriority=Speed  TableDataTypeStr=Inherit: Inherit from 'Table data'
      settings: InputPortMap=u0,u1,u2,u3,u4,u5,u6,u7,u8
  Interpolation Using Prelookup4 : Interpolation_n-D  NumberOfTableDimensions=5  Table=dp_WING_tip.CMx  ExtrapMethod=Clip  ValidIndexMayReachLast=on  NumSelectionDims=1  InternalRulePriority=Speed  TableDataTypeStr=Inherit: Inherit from 'Table data'
      settings: InputPortMap=u0,u1,u2,u3,u4,u5,u6,u7,u8
  Interpolation Using Prelookup5 : Interpolation_n-D  NumberOfTableDimensions=5  Table=dp_WING_tip.CMy  ExtrapMethod=Clip  ValidIndexMayReachLast=on  NumSelectionDims=1  InternalRulePriority=Speed  TableDataTypeStr=Inherit: Inherit from 'Table data'
      settings: InputPortMap=u0,u1,u2,u3,u4,u5,u6,u7,u8
  Interpolation Using Prelookup6 : Interpolation_n-D  NumberOfTableDimensions=5  Table=dp_WING_tip.CMz  ExtrapMethod=Clip  ValidIndexMayReachLast=on  NumSelectionDims=1  InternalRulePriority=Speed  TableDataTypeStr=Inherit: Inherit from 'Table data'
      settings: InputPortMap=u0,u1,u2,u3,u4,u5,u6,u7,u8
  WingRootPreLookup : Subsystem
  CD : Outport
  CS : Outport  Port=2
  CL : Outport  Port=3
  CMx : Outport  Port=4
  CMy : Outport  Port=5
  CMz : Outport  Port=6
  wires:
  Interpolation Using Prelookup6/1 -> CMz/1
  Interpolation Using Prelookup5/1 -> CMy/1
  Interpolation Using Prelookup4/1 -> CMx/1
  Interpolation Using Prelookup3/1 -> CL/1
  Interpolation Using Prelookup2/1 -> CS/1
  alpha/1 -> WingRootPreLookup/2(alpha)
  V_node/1 -> WingRootPreLookup/3(V_node)
  DEP_J/1 -> WingRootPreLookup/4(DEP_J)
  WingRootPreLookup/2(Out2) -> Interpolation Using Prelookup1/2, Interpolation Using Prelookup2/2, Interpolation Using Prelookup3/2, Interpolation Using Prelookup4/2, Interpolation Using Prelookup5/2, Interpolation Using Prelookup6/2
  WingRootPreLookup/6(Out7) -> Interpolation Using Prelookup1/6, Interpolation Using Prelookup2/6, Interpolation Using Prelookup3/6, Interpolation Using Prelookup4/6, Interpolation Using Prelookup5/6, Interpolation Using Prelookup6/6
  Interpolation Using Prelookup1/1 -> CD/1
  WingRootPreLookup/5(Out6) -> Interpolation Using Prelookup2/5, Interpolation Using Prelookup3/5, Interpolation Using Prelookup4/5, Interpolation Using Prelookup5/5, Interpolation Using Prelookup6/5, Interpolation Using Prelookup1/5
  WingRootPreLookup/4(Out4) -> Interpolation Using Prelookup1/4, Interpolation Using Prelookup2/4, Interpolation Using Prelookup3/4, Interpolation Using Prelookup4/4, Interpolation Using Prelookup5/4, Interpolation Using Prelookup6/4
  ail_defl/1 -> WingRootPreLookup/1(ail_defl)
  WingRootPreLookup/7(Out8) -> Interpolation Using Prelookup1/7, Interpolation Using Prelookup2/7, Interpolation Using Prelookup3/7, Interpolation Using Prelookup4/7, Interpolation Using Prelookup6/7, Interpolation Using Prelookup5/7
  WingRootPreLookup/1(Out1) -> Interpolation Using Prelookup1/1, Interpolation Using Prelookup2/1, Interpolation Using Prelookup3/1, Interpolation Using Prelookup4/1, Interpolation Using Prelookup5/1, Interpolation Using Prelookup6/1
  WingRootPreLookup/8(Out9) -> Interpolation Using Prelookup1/8, Interpolation Using Prelookup2/8, Interpolation Using Prelookup3/8, Interpolation Using Prelookup4/8, Interpolation Using Prelookup5/8, Interpolation Using Prelookup6/8
  WingRootPreLookup/3(Out3) -> Interpolation Using Prelookup1/3, Interpolation Using Prelookup2/3, Interpolation Using Prelookup3/3, Interpolation Using Prelookup4/3, Interpolation Using Prelookup5/3, Interpolation Using Prelookup6/3
  WingRootPreLookup/9(Out5) -> Interpolation Using Prelookup1/9, Interpolation Using Prelookup2/9, Interpolation Using Prelookup3/9, Interpolation Using Prelookup4/9, Interpolation Using Prelookup5/9, Interpolation Using Prelookup6/9

== system UNIFIER_3DOFsim/UNIFIER/Aerodynamics/HFM/Aero/WingForces/Left/Subsystem/CrossProduct ==
  r : Inport  Partition=on  PartitionDimension=2  PartitionWidth=1  PartitionOffset=0
  F : Inport  Port=2  Partition=on  PartitionDimension=2  PartitionWidth=1  PartitionOffset=0
  3x3 Cross Product : sharedutil/3x3 Cross Product  aMode=aMode
  CG : Constant  Value=xyz_cg
  Cast : DataTypeConversion  OutDataTypeStr=single  SaturateOnIntegerOverflow=off  RndMeth=Floor
  For Each : ForEach  DisableCoverage=on  SpecifiedNumIters=7
  Minus : Sum  Inputs=+-
  M : Outport  ConcatenationDimension=2
  wires:
  Cast/1 -> Minus/2
  Minus/1 -> 3x3 Cross Product/1
  CG/1 -> Cast/1
  3x3 Cross Product/1 -> M/1
  r/1 -> Minus/1
  F/1 -> 3x3 Cross Product/2

== system UNIFIER_3DOFsim/UNIFIER/Aerodynamics/HFM/Aero/WingForces/Left/Subsystem/w2b ==
  alpha : Inport  OutDataTypeStr=single  Partition=on  PartitionDimension=1  PartitionWidth=1  PartitionOffset=0
  Fw : Inport  Port=2  Partition=on  PartitionDimension=2  PartitionWidth=1  PartitionOffset=0
  Cast To Double : DataTypeConversion  OutDataTypeStr=double  SaturateOnIntegerOverflow=off  RndMeth=Floor
  Cast To Single : DataTypeConversion  OutDataTypeStr=single  SaturateOnIntegerOverflow=off  RndMeth=Floor
  Constant : Constant  Value=0  OutDataTypeStr=single
  Demux : Demux  Outputs=3
  Direction Cosine Matrix Body to Wind : aerolibtransform2/Direction Cosine Matrix Body to Wind
  For Each : ForEach  DisableCoverage=on  SpecifiedNumIters=7
  Matrix Multiply : Product  Multiplication=Matrix(*)
  Mux : Mux  Inputs=3
  Mux1 : Mux  Inputs=2
  Transpose : Math  Operator=transpose
  Unary Minus : UnaryMinus
  Unary Minus1 : UnaryMinus
  Fb : Outport  ConcatenationDimension=2
  wires:
  Cast To Double/1 -> Direction Cosine Matrix Body to Wind/1
  Cast To Single/1 -> Matrix Multiply/1
  Constant/1 -> Mux1/2
  Mux1/1 -> Cast To Double/1
  Transpose/1 -> Cast To Single/1
  Direction Cosine Matrix Body to Wind/1 -> Transpose/1
  Demux/3 -> Unary Minus1/1
  Unary Minus1/1 -> Mux/3
  Demux/2 -> Mux/2
  Unary Minus/1 -> Mux/1
  Demux/1 -> Unary Minus/1
  Mux/1 -> Matrix Multiply/2
  Matrix Multiply/1 -> Fb/1
  alpha/1 -> Mux1/1
  Fw/1 -> Demux/1

== system UNIFIER_3DOFsim/UNIFIER/Aerodynamics/HFM/Aero/WingForces/Left/WingRootForces/WingRootPreLookup ==
  flap_defl : Inport
  alpha : Inport  Port=2
  V_node : Inport  Port=3
  DEP_J : Inport  Port=4
  Constant8 : Constant  Value=0:4
  Prelookup : PreLookup  BreakpointsData=dp_WING_root.flap_defl  IndexSearchMethod=Linear search  BeginIndexSearchUsingPreviousIndexResult=on  UseLastBreakpoint=on
  Prelookup1 : PreLookup  BreakpointsData=dp_WING_root.alphas  IndexSearchMethod=Linear search  BeginIndexSearchUsingPreviousIndexResult=on  UseLastBreakpoint=on
  Prelookup2 : PreLookup  BreakpointsData=dp_WING_root.V  IndexSearchMethod=Linear search  BeginIndexSearchUsingPreviousIndexResult=on  UseLastBreakpoint=on
  Prelookup3 : PreLookup  BreakpointsData=dp_WING_root.DEP_J  IndexSearchMethod=Linear search  BeginIndexSearchUsingPreviousIndexResult=on  UseLastBreakpoint=on
  Out1 : Outport
  Out2 : Outport  Port=2
  Out3 : Outport  Port=3
  Out4 : Outport  Port=4
  Out6 : Outport  Port=5
  Out7 : Outport  Port=6
  Out8 : Outport  Port=7
  Out9 : Outport  Port=8
  Out5 : Outport  Port=9
  wires:
  Prelookup3/2 -> Out9/1
  Prelookup3/1 -> Out8/1
  Prelookup2/2 -> Out7/1
  Prelookup2/1 -> Out6/1
  DEP_J/1 -> Prelookup3/1
  V_node/1 -> Prelookup2/1
  flap_defl/1 -> Prelookup/1
  Prelookup1/1 -> Out3/1
  alpha/1 -> Prelookup1/1
  Prelookup/2 -> Out2/1
  Prelookup1/2 -> Out4/1
  Constant8/1 -> Out5/1
  Prelookup/1 -> Out1/1

== system UNIFIER_3DOFsim/UNIFIER/Aerodynamics/HFM/Aero/WingForces/Left/WingTipForces/WingRootPreLookup ==
  ail_defl : Inport
  alpha : Inport  Port=2
  V_node : Inport  Port=3
  DEP_J : Inport  Port=4
  Constant8 : Constant  Value=0:1
  Prelookup : PreLookup  BreakpointsData=dp_WING_tip.ail_defl  IndexSearchMethod=Linear search  BeginIndexSearchUsingPreviousIndexResult=on  UseLastBreakpoint=on
  Prelookup1 : PreLookup  BreakpointsData=dp_WING_tip.alphas  IndexSearchMethod=Linear search  BeginIndexSearchUsingPreviousIndexResult=on  UseLastBreakpoint=on
  Prelookup2 : PreLookup  BreakpointsData=dp_WING_tip.V  IndexSearchMethod=Linear search  BeginIndexSearchUsingPreviousIndexResult=on  UseLastBreakpoint=on
  Prelookup3 : PreLookup  BreakpointsData=dp_WING_tip.DEP_J  IndexSearchMethod=Linear search  BeginIndexSearchUsingPreviousIndexResult=on  UseLastBreakpoint=on
  Out1 : Outport
  Out2 : Outport  Port=2
  Out3 : Outport  Port=3
  Out4 : Outport  Port=4
  Out6 : Outport  Port=5
  Out7 : Outport  Port=6
  Out8 : Outport  Port=7
  Out9 : Outport  Port=8
  Out5 : Outport  Port=9
  wires:
  Prelookup3/2 -> Out9/1
  Prelookup3/1 -> Out8/1
  Prelookup2/2 -> Out7/1
  Prelookup2/1 -> Out6/1
  DEP_J/1 -> Prelookup3/1
  V_node/1 -> Prelookup2/1
  ail_defl/1 -> Prelookup/1
  Prelookup1/1 -> Out3/1
  alpha/1 -> Prelookup1/1
  Prelookup/2 -> Out2/1
  Prelookup1/2 -> Out4/1
  Constant8/1 -> Out5/1
  Prelookup/1 -> Out1/1

== system UNIFIER_3DOFsim/UNIFIER/Aerodynamics/HFM/Aero/WingForces/Right/Subsystem/CrossProduct ==
  r : Inport  Partition=on  PartitionDimension=2  PartitionWidth=1  PartitionOffset=0
  F : Inport  Port=2  Partition=on  PartitionDimension=2  PartitionWidth=1  PartitionOffset=0
  3x3 Cross Product : sharedutil/3x3 Cross Product  aMode=aMode
  CG : Constant  Value=xyz_cg
  Cast : DataTypeConversion  OutDataTypeStr=single  SaturateOnIntegerOverflow=off  RndMeth=Floor
  For Each : ForEach  DisableCoverage=on  SpecifiedNumIters=7
  Minus : Sum  Inputs=+-
  M : Outport  ConcatenationDimension=2
  wires:
  Cast/1 -> Minus/2
  Minus/1 -> 3x3 Cross Product/1
  CG/1 -> Cast/1
  3x3 Cross Product/1 -> M/1
  r/1 -> Minus/1
  F/1 -> 3x3 Cross Product/2

== system UNIFIER_3DOFsim/UNIFIER/Aerodynamics/HFM/Aero/WingForces/Right/Subsystem/w2b ==
  alpha : Inport  OutDataTypeStr=single  Partition=on  PartitionDimension=1  PartitionWidth=1  PartitionOffset=0
  Fw : Inport  Port=2  Partition=on  PartitionDimension=2  PartitionWidth=1  PartitionOffset=0
  Cast To Double : DataTypeConversion  OutDataTypeStr=double  SaturateOnIntegerOverflow=off  RndMeth=Floor
  Cast To Single : DataTypeConversion  OutDataTypeStr=single  SaturateOnIntegerOverflow=off  RndMeth=Floor
  Constant : Constant  Value=0  OutDataTypeStr=single
  Demux : Demux  Outputs=3
  Direction Cosine Matrix Body to Wind : aerolibtransform2/Direction Cosine Matrix Body to Wind
  Display : Display
  Display1 : Display
  For Each : ForEach  DisableCoverage=on  SpecifiedNumIters=7
  Matrix Multiply : Product  Multiplication=Matrix(*)
  Mux : Mux  Inputs=3
  Mux1 : Mux  Inputs=2
  Transpose : Math  Operator=transpose
  Unary Minus : UnaryMinus
  Unary Minus1 : UnaryMinus
  Fb : Outport  ConcatenationDimension=2
  wires:
  Cast To Double/1 -> Direction Cosine Matrix Body to Wind/1
  Cast To Single/1 -> Matrix Multiply/1
  Constant/1 -> Mux1/2
  Mux1/1 -> Cast To Double/1
  Transpose/1 -> Cast To Single/1
  Direction Cosine Matrix Body to Wind/1 -> Transpose/1
  Demux/3 -> Unary Minus1/1
  Unary Minus1/1 -> Mux/3
  Demux/2 -> Mux/2
  Unary Minus/1 -> Mux/1
  Demux/1 -> Unary Minus/1
  Mux/1 -> Matrix Multiply/2
  Matrix Multiply/1 -> Fb/1
  alpha/1 -> Mux1/1, Display/1
  Fw/1 -> Demux/1, Display1/1
